simulink model "EReg_v2_N2O"  (R2025b)
settings: Solver=FixedStepDiscrete  StartTime=0.0  StopTime=Sim_Duration  FixedStep=Ts_sim  RelTol=1e-3
undefined symbols (not defined in the file): A_3, backlash_init, Cd_3, cv_N2, DiscIntNeverNeededParam, gamma_N2, K_v_4, Kv_1_max, m_1_0, m_N2O_0, m_N2tank_0, n2o_lut, Pst, R_N2, rho_1_0, rhost, T_0_N2, Ts_ctrl, Ts_sim, Tst, U_n2o_0, V_1, V_2
settings Model: Creator=ethan  LastModifiedBy=ethan
settings DebuggingCC: AlgebraicLoopMsg=error

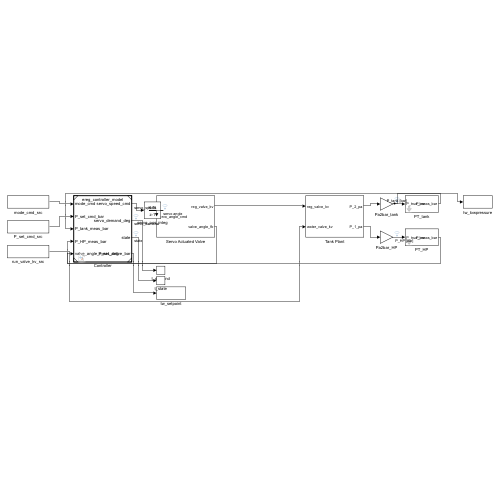
[thumbnail: Simulink's stored preview of the top-level diagram]
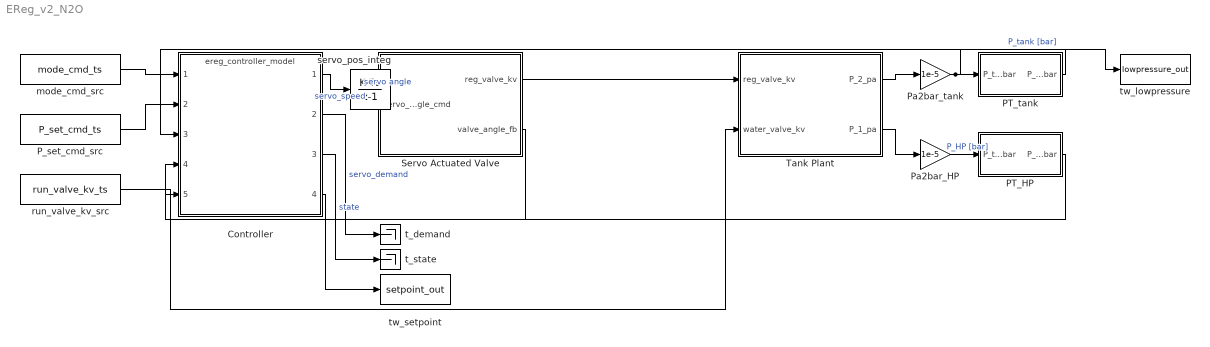
== system EReg_v2_N2O ==
  Controller : ModelReference  ModelNameDialog=ereg_controller_model  SimulationMode=Normal  ModelReferenceVersion=1.1
  PT_HP : Subsystem  mask{Ts_pt=0, noise_std_bar=0, quant_lsb_bar=0, seed=0}
      mask prompts: Ts_pt "PT sample time [s]"; noise_std_bar "Noise std [bar]"; quant_lsb_bar "Quantization LSB [bar]"; seed "Noise seed"
      mask help:
      | Pressure transducer placeholder (pure passthrough).
      | Upgrade recipe: inside, insert ZOH (Ts_pt) -> add Random Number (seed, noise_std_bar) -> Quantizer (quant_lsb_bar). Mask params are declared but unused until then.
  PT_tank : Subsystem  mask{Ts_pt=0, noise_std_bar=0, quant_lsb_bar=0, seed=0}
      mask prompts: Ts_pt "PT sample time [s]"; noise_std_bar "Noise std [bar]"; quant_lsb_bar "Quantization LSB [bar]"; seed "Noise seed"
      mask help:
      | Pressure transducer placeholder (pure passthrough).
      | Upgrade recipe: inside, insert ZOH (Ts_pt) -> add Random Number (seed, noise_std_bar) -> Quantizer (quant_lsb_bar). Mask params are declared but unused until then.
  P_set_cmd_src : FromWorkspace  VariableName=P_set_cmd_ts  SampleTime=Ts_sim  ZeroCross=off  OutputAfterFinalValue=Holding final value
  Pa2bar_HP : Gain  Gain=1e-5
  Pa2bar_tank : Gain  Gain=1e-5
  Servo Actuated Valve : Subsystem
  Tank Plant : Subsystem
  mode_cmd_src : FromWorkspace  VariableName=mode_cmd_ts  SampleTime=Ts_sim  Interpolate=off  ZeroCross=off  OutputAfterFinalValue=Holding final value
  run_valve_kv_src : FromWorkspace  VariableName=run_valve_kv_ts  SampleTime=Ts_sim  ZeroCross=off  OutputAfterFinalValue=Holding final value
  servo_pos_integ : DiscreteIntegrator  SampleTime=Ts_ctrl  ICPrevOutput=DiscIntNeverNeededParam  ICPrevScaledInput=DiscIntNeverNeededParam
  t_demand : Terminator
  t_state : Terminator
  tw_lowpressure : ToWorkspace  VariableName=lowpressure_out  SaveFormat=Timeseries  SampleTime=-1
  tw_setpoint : ToWorkspace  VariableName=setpoint_out  SaveFormat=Timeseries  SampleTime=-1
  wires:
  mode_cmd_src/1 -> Controller/1
  P_set_cmd_src/1 -> Controller/2
  Controller/1 -> servo_pos_integ/1  "servo_speed"
  servo_pos_integ/1 -> Servo Actuated Valve/1(servo_angle_cmd)  "servo angle"
  Controller/2 -> t_demand/1  "servo_demand"
  Controller/3 -> t_state/1  "state"
  Controller/4 -> tw_setpoint/1
  Servo Actuated Valve/1(reg_valve_kv) -> Tank Plant/1(reg_valve_kv)
  run_valve_kv_src/1 -> Tank Plant/2(water_valve_kv)
  Tank Plant/1(P_2_pa) -> Pa2bar_tank/1
  Pa2bar_tank/1 -> PT_tank/1(P_true_bar), tw_lowpressure/1  "P_tank [bar]"
  PT_tank/1(P_meas_bar) -> Controller/3
  Tank Plant/2(P_1_pa) -> Pa2bar_HP/1
  Pa2bar_HP/1 -> PT_HP/1(P_true_bar)  "P_HP [bar]"
  PT_HP/1(P_meas_bar) -> Controller/4
  Servo Actuated Valve/2(valve_angle_fb) -> Controller/5

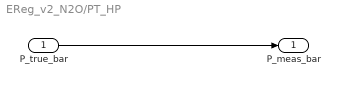
== system EReg_v2_N2O/PT_HP ==
  P_true_bar : Inport
  P_meas_bar : Outport
  wires:
  P_true_bar/1 -> P_meas_bar/1

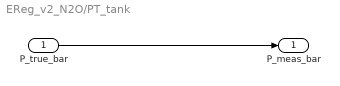
== system EReg_v2_N2O/PT_tank ==
  P_true_bar : Inport
  P_meas_bar : Outport
  wires:
  P_true_bar/1 -> P_meas_bar/1

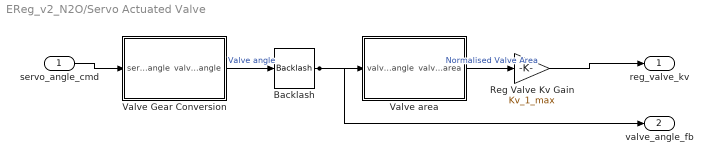
== system EReg_v2_N2O/Servo Actuated Valve ==
  servo_angle_cmd : Inport
  Backlash : Backlash  BacklashWidth=backlash_width  InitialOutput=backlash_init
  Reg Valve Kv Gain : Gain  Gain=Kv_1_max
  Valve Gear Conversion : MATLAB Function  TreatAsAtomicUnit=on
  Valve area : MATLAB Function  TreatAsAtomicUnit=on
  reg_valve_kv : Outport
  valve_angle_fb : Outport  Port=2
  wires:
  servo_angle_cmd/1 -> Valve Gear Conversion/1(servo_angle)
  Valve Gear Conversion/1(valve_angle) -> Backlash/1  "Valve angle"
  Backlash/1 -> Valve area/1(valve_angle), valve_angle_fb/1
  Valve area/1(valve_area) -> Reg Valve Kv Gain/1  "Normalised Valve Area"
  Reg Valve Kv Gain/1 -> reg_valve_kv/1

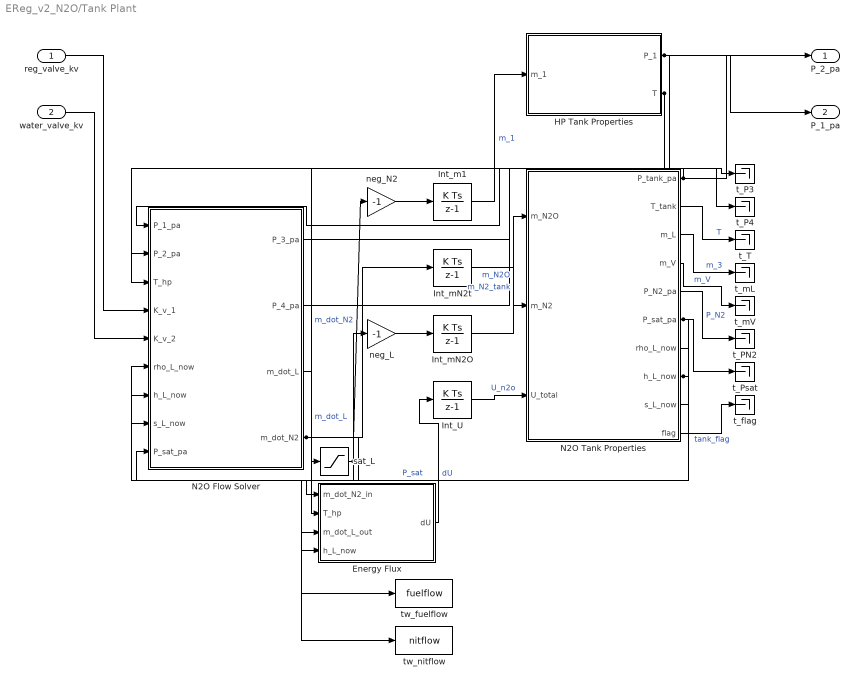
== system EReg_v2_N2O/Tank Plant ==
  reg_valve_kv : Inport
  water_valve_kv : Inport  Port=2
  Energy Flux : MATLAB Function  TreatAsAtomicUnit=on
  HP Tank Properties : MATLAB Function  TreatAsAtomicUnit=on
  Int_U : DiscreteIntegrator  InitialCondition=U_n2o_0  SampleTime=Ts_sim  ICPrevOutput=DiscIntNeverNeededParam  ICPrevScaledInput=DiscIntNeverNeededParam
  Int_m1 : DiscreteIntegrator  InitialCondition=m_1_0  SampleTime=Ts_sim  ICPrevOutput=DiscIntNeverNeededParam  ICPrevScaledInput=DiscIntNeverNeededParam
  Int_mN2O : DiscreteIntegrator  InitialCondition=m_N2O_0  SampleTime=Ts_sim  ICPrevOutput=DiscIntNeverNeededParam  ICPrevScaledInput=DiscIntNeverNeededParam
  Int_mN2t : DiscreteIntegrator  InitialCondition=m_N2tank_0  SampleTime=Ts_sim  ICPrevOutput=DiscIntNeverNeededParam  ICPrevScaledInput=DiscIntNeverNeededParam
  N2O Flow Solver : MATLAB Function  TreatAsAtomicUnit=on
  N2O Tank Properties : MATLAB Function  TreatAsAtomicUnit=on
  neg_L : Gain  Gain=-1
  neg_N2 : Gain  Gain=-1
  sat_L : Saturate  UpperLimit=inf  LowerLimit=0
  t_P3 : Terminator
  t_P4 : Terminator
  t_PN2 : Terminator
  t_Psat : Terminator
  t_T : Terminator
  t_flag : Terminator
  t_mL : Terminator
  t_mV : Terminator
  tw_fuelflow : ToWorkspace  VariableName=fuelflow  SaveFormat=Timeseries  SampleTime=-1
  tw_nitflow : ToWorkspace  VariableName=nitflow  SaveFormat=Timeseries  SampleTime=-1
  P_2_pa : Outport
  P_1_pa : Outport  Port=2
  wires:
  Int_m1/1 -> HP Tank Properties/1(m_1)  "m_1"
  HP Tank Properties/1(P_1) -> N2O Flow Solver/1(P_1_pa), P_1_pa/1
  HP Tank Properties/2(T) -> N2O Flow Solver/3(T_hp), Energy Flux/2(T_hp)
  Int_mN2O/1 -> N2O Tank Properties/1(m_N2O)  "m_N2O"
  Int_mN2t/1 -> N2O Tank Properties/2(m_N2)  "m_N2_tank"
  Int_U/1 -> N2O Tank Properties/3(U_total)  "U_n2o"
  N2O Tank Properties/1(P_tank_pa) -> N2O Flow Solver/2(P_2_pa), P_2_pa/1
  N2O Tank Properties/2(T_tank) -> t_T/1  "T"
  N2O Tank Properties/3(m_L) -> t_mL/1  "m_3"
  N2O Tank Properties/4(m_V) -> t_mV/1  "m_V"
  N2O Tank Properties/5(P_N2_pa) -> t_PN2/1  "P_N2"
  N2O Tank Properties/6(P_sat_pa) -> t_Psat/1, N2O Flow Solver/9(P_sat_pa)  "P_sat"
  N2O Tank Properties/7(rho_L_now) -> N2O Flow Solver/6(rho_L_now)
  N2O Tank Properties/8(h_L_now) -> N2O Flow Solver/7(h_L_now), Energy Flux/4(h_L_now)
  N2O Tank Properties/9(s_L_now) -> N2O Flow Solver/8(s_L_now)
  N2O Tank Properties/10(flag) -> t_flag/1  "tank_flag"
  reg_valve_kv/1 -> N2O Flow Solver/4(K_v_1)
  water_valve_kv/1 -> N2O Flow Solver/5(K_v_2)
  N2O Flow Solver/1(P_3_pa) -> t_P3/1
  N2O Flow Solver/2(P_4_pa) -> t_P4/1
  N2O Flow Solver/3(m_dot_L) -> sat_L/1  "m_dot_L"
  N2O Flow Solver/4(m_dot_N2) -> neg_N2/1, Int_mN2t/1, tw_nitflow/1, Energy Flux/1(m_dot_N2_in)  "m_dot_N2"
  neg_N2/1 -> Int_m1/1
  sat_L/1 -> neg_L/1, tw_fuelflow/1, Energy Flux/3(m_dot_L_out)
  neg_L/1 -> Int_mN2O/1
  Energy Flux/1(dU) -> Int_U/1  "dU"

== matlab function EReg_v2_N2O/Servo Actuated Valve/Valve area ==
  data: valve_angle input; valve_area output
function valve_area = fcn(valve_angle)
%     % BUG RECREATION: hardware has angle convention inverted vs sim
%     % Sim convention was: 0°=closed, 90°=open
%     % Hardware reality:   0°=open,   90°=closed
%     % Equivalent: feed (90 - valve_angle) through the same polynomial
%     inverted_angle = 90 - valve_angle;
%     inverted_angle = inverted_angle - 5;  % keep the same deadband
%     if inverted_angle < 0
%         valve_area = 0;
%     else
%         valve_area = 1.1*((5*10^-6)*inverted_angle^3 - 0.0006*inverted_angle^2 + 0.0278*inverted_angle);
%     end
% end

valve_angle = valve_angle - 5; %Account for first part of rotation where valve doesn't open at all
if valve_angle < 0
    valve_area = 0;
else
    valve_area = 1.1*((5*10^-6)*valve_angle^3 - 0.0006*valve_angle^2 + 0.0278*valve_angle); %calculate normalised valve area
end

== matlab function EReg_v2_N2O/Tank Plant/N2O Tank Properties ==
  data: m_N2O input; P_tank_pa output; m_N2 input; U_total input; T_tank output; m_L output; m_V output; P_N2_pa output; P_sat_pa output; rho_L_now output; h_L_now output; s_L_now output; flag output; V_2 parameter; n2o_lut parameter; R_N2 parameter; cv_N2 parameter
function [P_tank_pa, T_tank, m_L, m_V, P_N2_pa, P_sat_pa, rho_L_now, h_L_now, s_L_now, flag] = ...
    n2o_tank_properties(m_N2O, m_N2, U_total, V_2, n2o_lut, R_N2, cv_N2)
%N2O_TANK_PROPERTIES Equilibrium two-phase N2O tank with N2 supercharge.
%
% State: total N2O mass, N2 pad mass, total internal energy (adiabatic walls).
% Assumes full thermodynamic equilibrium at one temperature T: saturated N2O
% liquid + vapor sharing the ullage with ideal-gas N2 (Dalton). Solves T by
% bisection on the energy closure:
%   m_V(T)  = rho_V*(V - m_N2O/rho_L)/(1 - rho_V/rho_L)   (volume closure)
%   U_calc(T) = m_L*u_L + m_V*u_V + m_N2*cv_N2*T           (energy closure)
% U_calc is monotone increasing in T over the saturation dome.
% flag: 0 ok, 1 phase-boundary clamp hit, 2 T pinned at LUT range edge.
%#codegen

Tlo = n2o_lut.T(1) + 0.25;
Thi = n2o_lut.T(end) - 0.25;
flag = 0;

for i = 1:55
    Tm = 0.5 * (Tlo + Thi);
    if u_closure(Tm, m_N2O, m_N2, V_2, n2o_lut, cv_N2) > U_total
        Thi = Tm;
    else
        Tlo = Tm;
    end
end
T_tank = 0.5 * (Tlo + Thi);
if T_tank < n2o_lut.T(1) + 0.5 || T_tank > n2o_lut.T(end) - 0.5
    flag = 2;
end

[~, m_V, m_L, clamped] = u_closure(T_tank, m_N2O, m_N2, V_2, n2o_lut, cv_N2);
if clamped
    flag = max(flag, 1);
end

rho_L_now = interp1(n2o_lut.T, n2o_lut.rho_L, T_tank);
P_sat_pa  = interp1(n2o_lut.T, n2o_lut.P, T_tank);
h_L_now   = interp1(n2o_lut.T, n2o_lut.h_L, T_tank);
s_L_now   = interp1(n2o_lut.T, n2o_lut.s_L, T_tank);

V_ull = V_2 - m_L / rho_L_now;
V_ull = max(V_ull, 1e-9);
P_N2_pa = m_N2 * R_N2 * T_tank / V_ull;
P_tank_pa = P_sat_pa + P_N2_pa;
end

function [Ucalc, m_V, m_L, clamped] = u_closure(T, m_N2O, m_N2, V_2, n2o_lut, cv_N2)
rhoL = interp1(n2o_lut.T, n2o_lut.rho_L, T);
rhoV = interp1(n2o_lut.T, n2o_lut.rho_V, T);
m_V_raw = rhoV * (V_2 - m_N2O / rhoL) / (1 - rhoV / rhoL);
m_V = min(max(m_V_raw, 0), m_N2O);
clamped = (m_V ~= m_V_raw);
m_L = m_N2O - m_V;
Ucalc = m_L * interp1(n2o_lut.T, n2o_lut.u_L, T) + m_V * interp1(n2o_lut.T, n2o_lut.u_V, T) ...
    + m_N2 * cv_N2 * T;
end

== matlab function EReg_v2_N2O/Tank Plant/HP Tank Properties ==
  data: m_1 input; P_1 output; T output; V_1 parameter; T_0_N2 parameter; rho_1_0 parameter; gamma_N2 parameter; R_N2 parameter
function [P_1, T] = hp_tank_properties(m_1, V_1, T_0_N2, rho_1_0, gamma_N2, R_N2)
%HP_TANK_PROPERTIES HP nitrogen bottle state (adiabatic blowdown, ideal gas).
% Same law as v1's Gas Volume Properties, HP side only.
%#codegen
rho_1 = m_1 / V_1;
T = T_0_N2 * (rho_1 / rho_1_0)^(gamma_N2 - 1);
P_1 = rho_1 * R_N2 * T;
end

== matlab function EReg_v2_N2O/Tank Plant/N2O Flow Solver ==
  data: P_1_pa input; P_3_pa output; P_2_pa input; T_hp input; K_v_1 input; K_v_2 input; rho_L_now input; h_L_now input; s_L_now input; P_sat_pa input; P_4_pa output; m_dot_L output; m_dot_N2 output; n2o_lut parameter; K_v_4 parameter; Cd_3 parameter; A_3 parameter; R_N2 parameter; Tst parameter; rhost parameter; Pst parameter
function [P_3_pa, P_4_pa, m_dot_L, m_dot_N2] = n2o_flow_solver( ...
    P_1_pa, P_2_pa, T_hp, K_v_1, K_v_2, rho_L_now, h_L_now, s_L_now, P_sat_pa, ...
    n2o_lut, K_v_4, Cd_3, A_3, R_N2, Tst, rhost, Pst)
%N2O_FLOW_SOLVER Component flows for the N2O variant.
%
% Gas side: verbatim v1 physics - solve P_4 between the regulator valve
% (choked/non-choked ISA Kv gas flow from the HP bottle) and the check valve
% into the tank ullage.
% Liquid side: solve P_3 between the run valve (Kv liquid flow, live N2O
% density) and a Dyer/NHNE injector orifice to atmosphere:
%   m_SPI = Cd*A*sqrt(2*rho_L*dP)
%   m_HEM = Cd*A*rho_2*sqrt(2*(h_1 - h_2)),  state 2 = isentropic to P_atm
%   m_dot = (k*m_SPI + m_HEM)/(1+k),  k = sqrt((P_3-P_atm)/(P_sat-P_atm))
% Supercharge (P_3 >> P_sat) drives k up -> SPI-dominated, as physics demands.
%#codegen

MAX_ITER = 60;
TOLERANCE = 1e-7;
h = 1e-6;
P_atm_pa = 101325;

P_1 = P_1_pa * 1e-5;
P_2 = P_2_pa * 1e-5;
SG = rho_L_now / 1000.0;

% --- Liquid side: P_3 between run valve and Dyer orifice ---
liquid_error_fun = @(p3) (calc_m_dot_valve(p3, P_2, K_v_2, rho_L_now, SG) - ...
    calc_m_dot_dyer(p3, P_atm_pa, Cd_3, A_3, rho_L_now, h_L_now, s_L_now, P_sat_pa, n2o_lut));
x0_P3 = max(P_2 - 0.5, 1.0);
P_3_bar = newton_solver(liquid_error_fun, x0_P3, MAX_ITER, TOLERANCE, h);
% robustness: bisection fallback if Newton wandered (kinks at the flash boundary)
if ~isfinite(P_3_bar) || abs(liquid_error_fun(P_3_bar)) > 1e-4
    P_3_bar = bisect(liquid_error_fun, P_atm_pa * 1e-5, max(P_2, 1.0) + 1.0, 80);
end

% --- Gas side: P_4 between regulator valve and check valve (v1 verbatim) ---
gas_error_fun = @(p4) (calc_m_dot_c(p4, P_1, K_v_1, rhost, T_hp, Pst, R_N2, Tst) - ...
    calc_m_dot_d(p4, P_2, K_v_4, rhost, T_hp, Pst, R_N2, Tst));
x0_P4 = 1.0;
P_4_bar = newton_solver(gas_error_fun, x0_P4, MAX_ITER, TOLERANCE, h);

P_3_pa = P_3_bar * 1e5;
P_4_pa = P_4_bar * 1e5;
m_dot_L  = calc_m_dot_valve(P_3_bar, P_2, K_v_2, rho_L_now, SG);
m_dot_N2 = calc_m_dot_c(P_4_bar, P_1, K_v_1, rhost, T_hp, Pst, R_N2, Tst);
end

% =========================================================================

function x_root = newton_solver(fun, x0, max_iter, tol, h)
x_root = x0;
for i = 1:max_iter
    f_val = fun(x_root);
    if abs(f_val) < tol
        return;
    end
    f_deriv = (fun(x_root + h) - f_val) / h;
    if abs(f_deriv) < 1e-10
        return;
    end
    x_new = x_root - f_val / f_deriv;
    if abs(x_new - x_root) < tol
        x_root = x_new;
        return;
    end
    x_root = x_new;
end
end

function x = bisect(fun, lo, hi, iters)
flo = fun(lo);
for i = 1:iters
    x = 0.5 * (lo + hi);
    fx = fun(x);
    if sign(fx) == sign(flo)
        lo = x; flo = fx;
    else
        hi = x;
    end
end
x = 0.5 * (lo + hi);
end

function m_dot = calc_m_dot_valve(P_3, P_2, K_v_2, rho_L, SG)
% Run valve, Kv liquid flow (v1 form, live density). Pressures in bar.
delta_P = P_2 - P_3;
Q = K_v_2 * (delta_P / SG) / sqrt(abs(delta_P / SG) + 1e-9);
m_dot = Q * rho_L * (1 / 3600);
end

function m_dot = calc_m_dot_dyer(P_3_bar, P_atm_pa, Cd, A, rho_L, h_1, s_1, P_sat_pa, n2o_lut)
% Dyer/NHNE orifice to atmosphere. Signed-SPI form keeps the solver smooth.
P_3_pa = P_3_bar * 1e5;
dP = P_3_pa - P_atm_pa;
m_spi = Cd * A * 2 * rho_L * dP / sqrt(abs(2 * rho_L * dP) + 1e-9);
if dP <= 0 || P_sat_pa <= P_atm_pa * 1.0001
    m_dot = m_spi;      % backflow or non-flashing regime: SPI only
    return;
end
% HEM branch: isentropic expansion to atmospheric saturation state
T_2 = interp1(n2o_lut.P, n2o_lut.T, P_atm_pa);
s_L2 = interp1(n2o_lut.T, n2o_lut.s_L, T_2);
s_V2 = interp1(n2o_lut.T, n2o_lut.s_V, T_2);
x_2 = (s_1 - s_L2) / (s_V2 - s_L2);
x_2 = min(max(x_2, 0), 1);
h_L2 = interp1(n2o_lut.T, n2o_lut.h_L, T_2);
h_V2 = interp1(n2o_lut.T, n2o_lut.h_V, T_2);
h_2 = h_L2 + x_2 * (h_V2 - h_L2);
rhoL2 = interp1(n2o_lut.T, n2o_lut.rho_L, T_2);
rhoV2 = interp1(n2o_lut.T, n2o_lut.rho_V, T_2);
rho_2 = 1 / ((1 - x_2) / rhoL2 + x_2 / rhoV2);
m_hem = Cd * A * rho_2 * sqrt(2 * max(h_1 - h_2, 0));
k = sqrt(dP / (P_sat_pa - P_atm_pa));
m_dot = (k * m_spi + m_hem) / (1 + k);
end

function m_dot_c = calc_m_dot_c(P_4, P_1, K_v_1, rhost, T, Pst, R_N2, Tst)
% Regulator valve (v1 verbatim). Pressures in bar.
Q_N = 0.0;
if (P_4 >= 0.528 * P_1)
    arg = (P_1 - P_4) * P_4 / (rhost * T);
    Q_N = K_v_1 * 514 * arg / sqrt(abs(arg) + 1e-9);
else
    Q_N = K_v_1 * 257 * P_1 / sqrt(abs(rhost * T) + 1e-9);
end
m_dot_c = Q_N * (Pst / (R_N2 * Tst)) * (1 / 3600);
end

function m_dot_d = calc_m_dot_d(P_4, P_2, K_v_4, rhost, T, Pst, R_N2, Tst)
% Check valve (v1 verbatim). Pressures in bar.
Q_N = 0.0;
if (P_2 >= 0.528 * P_4)
    arg = (P_4 - P_2) * P_2 / (rhost * T);
    Q_N = K_v_4 * 514 * arg / sqrt(abs(arg) + 1e-9);
else
    Q_N = K_v_4 * 257 * P_4 / sqrt(abs(rhost * T) + 1e-9);
end
m_dot_d = Q_N * (Pst / (R_N2 * Tst)) * (1 / 3600);
end

== matlab function EReg_v2_N2O/Tank Plant/Energy Flux ==
  data: m_dot_N2_in input; dU output; T_hp input; m_dot_L_out input; h_L_now input; cp_N2 parameter
function dU = n2o_energy_flux(m_dot_N2_in, T_hp, m_dot_L_out, h_L_now, cp_N2)
%N2O_ENERGY_FLUX Rate of change of the LP tank's total internal energy.
% Adiabatic walls: N2 enters at HP-line temperature carrying cp*T enthalpy;
% saturated liquid leaves carrying h_L. Must be fed the SAME clamped liquid
% flow that feeds the m_N2O integrator.
%#codegen
dU = m_dot_N2_in * cp_N2 * T_hp - m_dot_L_out * h_L_now;
end

== matlab function EReg_v2_N2O/Servo Actuated Valve/Valve Gear Conversion ==
  data: servo_angle input; valve_angle output
function valve_angle = fcn(servo_angle)

valve_angle = servo_angle/1.7; % check gear ratio with oscar
%valve_angle = servo_angle;
